simulink model "speed2"  (R2022b)
settings: Solver=VariableStepAuto  StartTime=0.0  StopTime=30  RelTol=1e-3
values from neighbouring files (symbols this model uses):
  Caf = 460.0    [VehCtrlMdelDictionary.sldd]    (also in trqvparameter.m = 460)
  Car = 440.0    [VehCtrlMdelDictionary.sldd]    (also in trqvparameter.m = 440)
  dwf = 1.2    [VehCtrlMdelDictionary.sldd]    (also in trqvparameter.m)
  Iz = 105.0    [VehCtrlMdelDictionary.sldd]    (also in trqvparameter.m = 105)
  Ki = 1.0    [VehCtrlMdelDictionary.sldd]    (also in trqvparameter.m = 20)
  Kp = 2.0    [VehCtrlMdelDictionary.sldd]    (also in trqvparameter.m = 30)
  lf = 0.761    [VehCtrlMdelDictionary.sldd]    (also in trqvparameter.m)
  lr = 0.831    [VehCtrlMdelDictionary.sldd]    (also in trqvparameter.m)
  m = 340.0    [VehCtrlMdelDictionary.sldd]    (also in trqvparameter.m = 340)
  Rt = 0.2    [VehCtrlMdelDictionary.sldd]    (also in trqvparameter.m)
libraries: simulink x12, Solver_SF x1
settings Model: Creator=12045  LastModifiedBy=12045

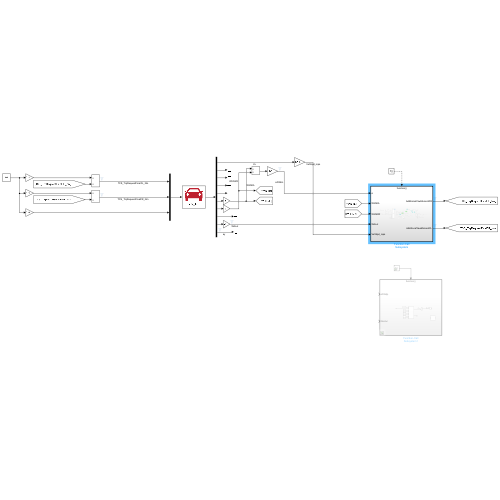
[thumbnail: Simulink's stored preview of the top-level diagram]
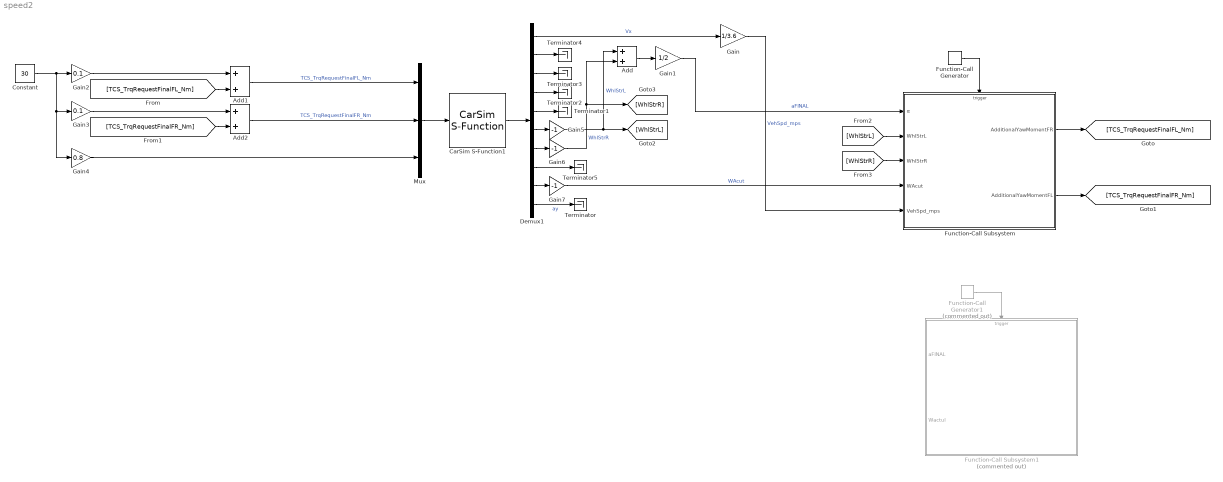
== system speed2 ==
  Add : Sum
  Add1 : Sum
  Add2 : Sum
  CarSim S-Function1 : Solver_SF/CarSim S-Function  Priority=1  SIMFILE=simfile.sim  Run_RTs=off  vs_state_ind=Run  StopMode_ind=Vehicle Model
  Constant : Constant  Value=30
  Demux1 : Demux  Outputs=10
  Function-Call Generator : simulink/Ports & Subsystems/Function-Call Generator  sample_time=0.01  numberOfIterations=1  DisallowWideOutput=off
  Function-Call Generator1 : simulink/Ports & Subsystems/Function-Call Generator  Commented=on  sample_time=0.01  numberOfIterations=1  DisallowWideOutput=off
  Function-Call Subsystem : Subsystem  TreatAsAtomicUnit=on
  Function-Call Subsystem1 : Subsystem  Commented=on  TreatAsAtomicUnit=on
  Gain : Gain  Gain=1/3.6
  Gain1 : Gain  Gain=1/2
  Gain2 : Gain  Gain=0.1
  Gain3 : Gain  Gain=0.1
  Gain4 : Gain  Gain=0.8
  Gain5 : Gain  Gain=-1
  Gain6 : Gain  Gain=-1
  Gain7 : Gain  Gain=-1
  Mux : Mux  Inputs=3
  Terminator{,1..5} (6 alike) : Terminator
  wires:
  Add2/1 -> Mux/2  "TCS_TrqRequestFinalFR_Nm"
  Add1/1 -> Mux/1  "TCS_TrqRequestFinalFL_Nm"
  Mux/1 -> CarSim S-Function1/1
  Function-Call Generator/1 -> Function-Call Subsystem/Trigger
  Gain6/1 -> Add/2, [WhlStrR]  "WhlStrR"
  Gain7/1 -> Function-Call Subsystem/4(WAcut)  "WAcut"
  Demux1/6 -> Gain5/1
  Demux1/7 -> Gain6/1
  Demux1/9 -> Gain7/1
  Gain5/1 -> [WhlStrL], Add/1  "WhlStrL"
  CarSim S-Function1/1 -> Demux1/1
  Demux1/10 -> Terminator/1  "ay"
  Demux1/1 -> Gain/1  "Vx"
  Add/1 -> Gain1/1
  Function-Call Subsystem/1(AdditionalYawMomentFR) -> [TCS_TrqRequestFinalFL_Nm]
  Function-Call Subsystem/2(AdditionalYawMomentFL) -> [TCS_TrqRequestFinalFR_Nm]
  [WhlStrL] -> Function-Call Subsystem/2(WhlStrL)
  [WhlStrR] -> Function-Call Subsystem/3(WhlStrR)
  Demux1/5 -> Terminator1/1
  Demux1/4 -> Terminator2/1
  Demux1/3 -> Terminator3/1
  Demux1/2 -> Terminator4/1
  Demux1/8 -> Terminator5/1
  Constant/1 -> Gain4/1, Gain3/1, Gain2/1
  Gain2/1 -> Add1/1
  [TCS_TrqRequestFinalFL_Nm] -> Add1/2
  Gain3/1 -> Add2/1
  [TCS_TrqRequestFinalFR_Nm] -> Add2/2
  Gain4/1 -> Mux/3
  Gain/1 -> Function-Call Subsystem/5(VehSpd_mps)  "VehSpd_mps"
  Gain1/1 -> Function-Call Subsystem/1(α)  "aFINAL"
  Function-Call Generator1/1 -> Function-Call Subsystem1/Trigger

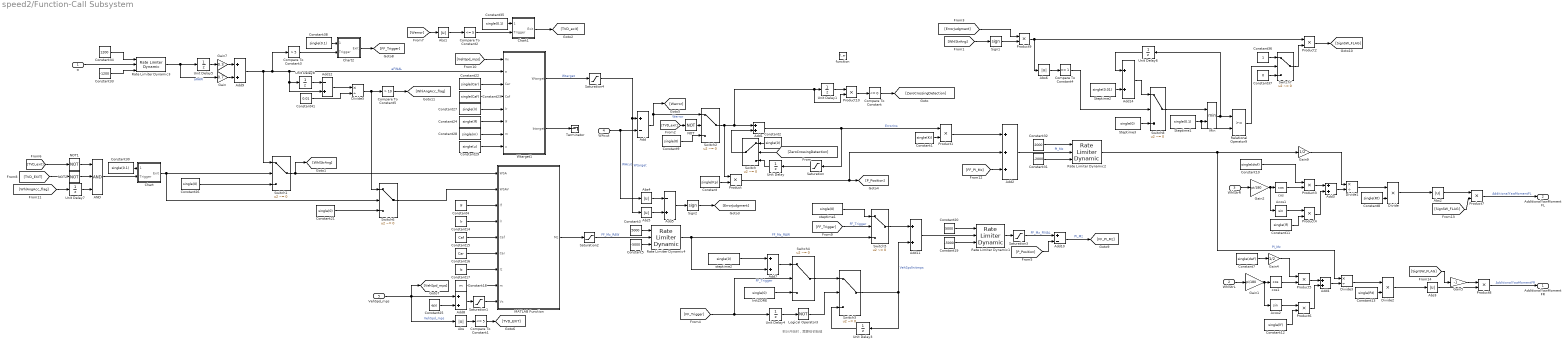
== system speed2/Function-Call Subsystem ==
  note: 积分开始时，需要给初始值
  α : Inport
  WhlStrL : Inport  Port=2
  WhlStrR : Inport  Port=3
  WAcut : Inport  Port=4
  VehSpd_mps : Inport  Port=5
  function : TriggerPort  TriggerType=function-call  VariantControl=(inherit)
  AND : Logic  Inputs=3  AllPortsSameDT=off  OutDataTypeStr=boolean
  Abs{,1..6} (7 alike) : Abs  SaturateOnIntegerOverflow=off
  Acos1 : Trigonometry
  Acos2 : Trigonometry
  Add : Sum  Inputs=+-
  Add{1,3..4,7..9,11,14} (8 alike) : Sum
  Add10 : Sum  Inputs=+-
  Add12 : Sum  Inputs=-+
  Add2 : Sum  Inputs=+++
  Add5 : Sum  Inputs=-+
  Chart : Stateflow chart  TreatAsAtomicUnit=on
  Chart1 : Stateflow chart  TreatAsAtomicUnit=on
  Chart2 : Stateflow chart  TreatAsAtomicUnit=on
  Compare To Constant : simulink/Logic and Bit Operations/Compare To Constant  relop=<=  const=0  OutDataTypeStr=boolean
  Compare To Constant1 : simulink/Logic and Bit Operations/Compare To Constant  relop=<=  const=5  OutDataTypeStr=boolean
  Compare To Constant2 : simulink/Logic and Bit Operations/Compare To Constant  relop=<=  const=5  OutDataTypeStr=boolean
  Compare To Constant3 : simulink/Logic and Bit Operations/Compare To Constant  relop=>  const=5  OutDataTypeStr=boolean
  Compare To Constant4 : simulink/Logic and Bit Operations/Compare To Constant  relop===  const=1  OutDataTypeStr=boolean
  Compare To Constant5 : simulink/Logic and Bit Operations/Compare To Constant  relop=>  const=10  OutDataTypeStr=boolean
  Constant : Constant  Value=single(Kp)
  Constant1 : Constant  Value=single(Ki)
  Constant10 : Constant  Value=single(dwf)
  Constant11 : Constant  Value=single(lf)
  Constant12 : Constant  Value=single(lf)
  Constant13 : Constant  Value=single(Rt)
  Constant14 : Constant  Value=lr
  Constant15 : Constant  Value=Caf
  Constant16 : Constant  Value=Car
  Constant17 : Constant  Value=Iz
  Constant18 : Constant  Value=m
  Constant19 : Constant  Value=-5000
  Constant{2,9,21,26} (4 alike) : Constant  Value=single(0)
  Constant20 : Constant  Value=5000
  Constant22 : Constant  Value=single(Car)
  Constant23 : Constant  Value=single(Caf)
  Constant24 : Constant  Value=single(lf)
  Constant25 : Constant  Value=eps
  Constant27 : Constant  Value=single(lr)
  Constant28 : Constant  Value=single(m)
  Constant29 : Constant  Value=single(u)
  Constant3 : Constant  Value=5000
  Constant30 : Constant  Value=single(0.1)
  Constant31 : Constant  Value=-2000
  Constant32 : Constant  Value=2000
  Constant33 : Constant  Value=-1200
  Constant34 : Constant  Value=1200
  Constant35 : Constant  Value=single(0.1)
  Constant36 : Constant
  Constant37 : Constant  Value=0
  Constant38 : Constant  Value=single(0.1)
  Constant4 : Constant  Value=lf
  Constant41 : Constant  Value=0.01
  Constant5 : Constant  Value=-5000
  Constant7 : Constant  Value=single(dwf)
  Constant8 : Constant  Value=single(Rt)
  Divide : Product  Inputs=**
  Divide1 : Product  Inputs=*/
  Divide2 : Product  Inputs=**
  Divide3 : Product  Inputs=*/
  Divide5 : Product  Inputs=*/
  Gain : Gain  Gain=0.7
  Gain1 : Gain  Gain=pi/180
  Gain2 : Gain  Gain=pi/180
  Gain4 : Gain  Gain=1/2
  Gain5 : Gain  Gain=-1
  Gain7 : Gain  Gain=0.3
  Gain9 : Gain  Gain=1/2
  InitZORE : Constant  Value=single(0)
  Logical Operator3 : Logic  Operator=NOT  AllPortsSameDT=off  OutDataTypeStr=boolean
  MATLAB Function : MATLAB Function  TreatAsAtomicUnit=on
  Min : MinMax  Inputs=2
  NOT : Logic  Operator=NOT  AllPortsSameDT=off  OutDataTypeStr=boolean
  NOT1 : Logic  Operator=NOT  AllPortsSameDT=off  OutDataTypeStr=boolean
  NOT2 : Logic  Operator=NOT  AllPortsSameDT=off  OutDataTypeStr=boolean
  Product{,1..10} (11 alike) : Product
  Rate Limiter Dynamic{1..4} (4 alike) : simulink/Discontinuities/Rate Limiter Dynamic
  Relational Operator9 : RelationalOperator  OutDataTypeStr=boolean  RndMeth=Simplest  InputSameDT=off
  Saturation : Saturate  UpperLimit=10  LowerLimit=-10
  Saturation1 : Saturate  UpperLimit=40  LowerLimit=0
  Saturation2 : Saturate  UpperLimit=5000  LowerLimit=-5000
  Saturation3 : Saturate  UpperLimit=300  LowerLimit=-300
  Saturation4 : Saturate  UpperLimit=50  LowerLimit=-50
  Sign1 : Signum
  Sign2 : Signum
  Steptime1 : Constant  Value=single(0.1)
  Steptime2 : Constant  Value=single(0.01)
  Steptime3 : Constant  Value=single(0)
  Switch{,1..8} (9 alike) : Switch  Criteria=u2 ~= 0  SaturateOnIntegerOverflow=off  InputSameDT=off
  Terminator : Terminator
  Unit Delay{,1,3..8} (8 alike) : UnitDelay  SampleTime=-1  HasFrameUpgradeWarning=on
  Wtarget1 : MATLAB Function  TreatAsAtomicUnit=on
  cos : Trigonometry  Operator=cos
  cos1 : Trigonometry  Operator=cos
  steptime1 : Constant  Value=single(0)
  steptime2 : Constant  Value=single(0)
  AdditionalYawMomentFR : Outport
  AdditionalYawMomentFL : Outport  Port=2
  wires:
  Wtarget1/1(Wtarget) -> Saturation4/1  "Wtarget"
  WAcut/1 -> Abs4/1, Add/2  "WAcut"
  Add/1 -> [Werror], Switch2/1  "Werror"
  Constant/1 -> Product/2
  Add1/1 -> Product1/1, Saturation/1  "ErrorIns"
  Constant1/1 -> Product1/2
  Product1/1 -> Add2/1
  Product/1 -> Add2/2, [P_Position]
  Saturation/1 -> Unit Delay/1
  Switch/1 -> Add1/2
  Constant2/1 -> Switch/1
  Unit Delay/1 -> Switch/3
  Compare To Constant/1 -> [ZeroCrossingDetection]
  [ZeroCrossingDetection] -> Switch/2
  Constant8/1 -> Divide/2
  Abs1/1 -> Compare To Constant2/1
  Switch2/1 -> Product10/2, Unit Delay1/1, Add1/1, Product/1
  [TVD_exit] -> NOT/1
  NOT/1 -> Switch2/2
  Constant9/1 -> Switch2/3
  WhlStrR/1 -> Gain2/1
  Gain2/1 -> Acos1/1, cos/1
  cos/1 -> Product3/2
  Constant10/1 -> Product3/1
  Product3/1 -> Add3/1
  Acos1/1 -> Product4/1
  Constant11/1 -> Product4/2
  Product4/1 -> Add3/2
  Add3/1 -> Divide1/2
  Divide1/1 -> Divide/1
  Divide/1 -> Abs2/1
  Divide3/1 -> Divide2/1
  Add4/1 -> Divide3/2
  Product6/1 -> Add4/2
  Constant12/1 -> Product6/2
  Acos2/1 -> Product6/1
  Product5/1 -> Add4/1
  Gain4/1 -> Product5/1
  cos1/1 -> Product5/2
  Constant7/1 -> Gain4/1
  Gain1/1 -> cos1/1, Acos2/1
  WhlStrL/1 -> Gain1/1
  Rate Limiter Dynamic2/1 -> Divide3/1, Gain9/1  "PI_Mz"
  Constant13/1 -> Divide2/2
  Divide2/1 -> Abs3/1
  Abs2/1 -> Product7/1
  Abs3/1 -> Product8/2
  Sign2/1 -> [ErrorJudgment]
  Sign1/1 -> Product9/2
  [ErrorJudgment] -> Product9/1
  Product9/1 -> Product2/1, Abs6/1
  Gain5/1 -> Product8/1
  Abs4/1 -> Add5/1
  Abs5/1 -> Add5/2
  Add5/1 -> Sign2/1
  Unit Delay1/1 -> Product10/1
  Product10/1 -> Compare To Constant/1
  Constant4/1 -> MATLAB Function/3(lf)
  Constant14/1 -> MATLAB Function/4(lr)
  Constant15/1 -> MATLAB Function/5(Caf)
  Constant16/1 -> MATLAB Function/6(Car)
  Constant17/1 -> MATLAB Function/7(Iz)
  Constant18/1 -> MATLAB Function/8(m)
  VehSpd_mps/1 -> Add8/1, Abs/1, [VehSpd_mps]  "VehSpd_mps"
  Switch1/1 -> [WhlStrAng], MATLAB Function/1(WSA)
  [WhlStrAng] -> Sign1/1
  Logical Operator3/1 -> Switch3/2
  steptime2/1 -> Add7/1
  Switch3/1 -> Add11/2, Unit Delay3/1  "VehSpdInitmps"
  Unit Delay4/1 -> Logical Operator3/1
  [FF_Trigger] -> Switch4/2, Unit Delay4/1  "FF_Trigger"
  Unit Delay3/1 -> Switch3/3
  Switch4/1 -> Switch3/1
  InitZORE/1 -> Switch4/3
  Add7/1 -> Switch4/1
  Add8/1 -> Saturation1/1
  Constant25/1 -> Add8/2
  Saturation1/1 -> MATLAB Function/9(Vx)
  [P_Position] -> Add10/2
  MATLAB Function/1(Mz) -> Saturation2/1
  Constant26/1 -> Switch1/3
  Rate Limiter Dynamic3/1 -> Unit Delay5/1, Gain/1  "aRAW"
  [TVD_exit] -> NOT1/1
  NOT1/1 -> AND/1
  [Werror] -> Abs1/1
  Rate Limiter Dynamic4/1 -> Add7/2, Switch5/3  "FF_Mz_RAW"
  Abs/1 -> Compare To Constant1/1
  Compare To Constant1/1 -> [TVD_EXIT]
  [TVD_EXIT] -> NOT2/1
  NOT2/1 -> AND/2
  Chart/1(Exit) -> Switch6/2, Switch1/2
  [FF_Trigger] -> Switch5/2  "FF_Trigger"
  Switch5/1 -> Add11/1
  steptime1/1 -> Switch5/1
  Add11/1 -> Rate Limiter Dynamic1/2
  Constant19/1 -> Rate Limiter Dynamic1/3
  Rate Limiter Dynamic1/1 -> Saturation3/1
  Constant20/1 -> Rate Limiter Dynamic1/1
  Saturation3/1 -> Add10/1  "FF_Mz_FINAL"
  Constant21/1 -> Switch6/3
  Switch6/1 -> MATLAB Function/2(WSAV)
  Constant22/1 -> Wtarget1/3(Car)
  Constant28/1 -> Wtarget1/7(m)
  Constant27/1 -> Wtarget1/5(lr)
  Constant29/1 -> Wtarget1/8(u)
  Constant24/1 -> Wtarget1/6(lf)
  Constant23/1 -> Wtarget1/4(Caf)
  [VehSpd_mps] -> Wtarget1/1(Vx)
  Wtarget1/2(btarget) -> Terminator/1
  Saturation4/1 -> Abs5/1, Add/1  "Wtarget"
  AND/1 -> Chart/2(Trigger)
  Constant30/1 -> Chart/1(CountTime)
  Constant32/1 -> Rate Limiter Dynamic2/1
  Constant31/1 -> Rate Limiter Dynamic2/3
  Add2/1 -> Rate Limiter Dynamic2/2  "PI_Mz"
  Unit Delay5/1 -> Gain7/1
  Add9/1 -> Compare To Constant3/1, Add12/2, Unit Delay8/1, Wtarget1/2(a), Switch1/1  "aFINAL"
  Gain/1 -> Add9/2
  Gain7/1 -> Add9/1
  α/1 -> Rate Limiter Dynamic3/2
  Constant33/1 -> Rate Limiter Dynamic3/3
  Constant34/1 -> Rate Limiter Dynamic3/1
  Product7/1 -> AdditionalYawMomentFL/1  "AdditionalYawMomentFL"
  Product8/1 -> AdditionalYawMomentFR/1  "AdditionalYawMomentFR"
  Abs6/1 -> Compare To Constant4/1
  Relational Operator9/1 -> Switch7/2
  Switch7/1 -> Product2/2
  Constant36/1 -> Switch7/1
  Constant37/1 -> Switch7/3
  Min/1 -> Relational Operator9/1, Unit Delay6/1
  Compare To Constant4/1 -> Switch8/2
  Add14/1 -> Switch8/1
  Unit Delay6/1 -> Add14/1
  Steptime3/1 -> Switch8/3
  Switch8/1 -> Min/1
  Steptime2/1 -> Add14/2
  Steptime1/1 -> Relational Operator9/2, Min/2
  [FF_PI_Mz] -> Add2/3
  Product2/1 -> [SignSW_FLAG]
  [SignSW_FLAG] -> Product7/2
  [SignSW_FLAG] -> Gain5/1
  Gain9/1 -> Divide1/1
  Constant35/1 -> Chart1/1(CountTime)
  Compare To Constant2/1 -> Chart1/2(Trigger)
  Chart1/1(Exit) -> [TVD_exit]
  Compare To Constant3/1 -> Chart2/2(Trigger)
  Constant38/1 -> Chart2/1(CountTime)
  Chart2/1(Exit) -> [FF_Trigger]
  Add10/1 -> [FF_PI_Mz]  "PI_Mz"
  Compare To Constant5/1 -> [WhlAngAcc_flag]
  [WhlAngAcc_flag] -> Unit Delay7/1
  Unit Delay7/1 -> AND/3
  Constant41/1 -> Divide5/2
  Add12/1 -> Divide5/1
  Unit Delay8/1 -> Add12/1
  Divide5/1 -> Switch6/1, Compare To Constant5/1
  Saturation2/1 -> Rate Limiter Dynamic4/2  "FF_Mz_RAW"
  Constant3/1 -> Rate Limiter Dynamic4/1
  Constant5/1 -> Rate Limiter Dynamic4/3

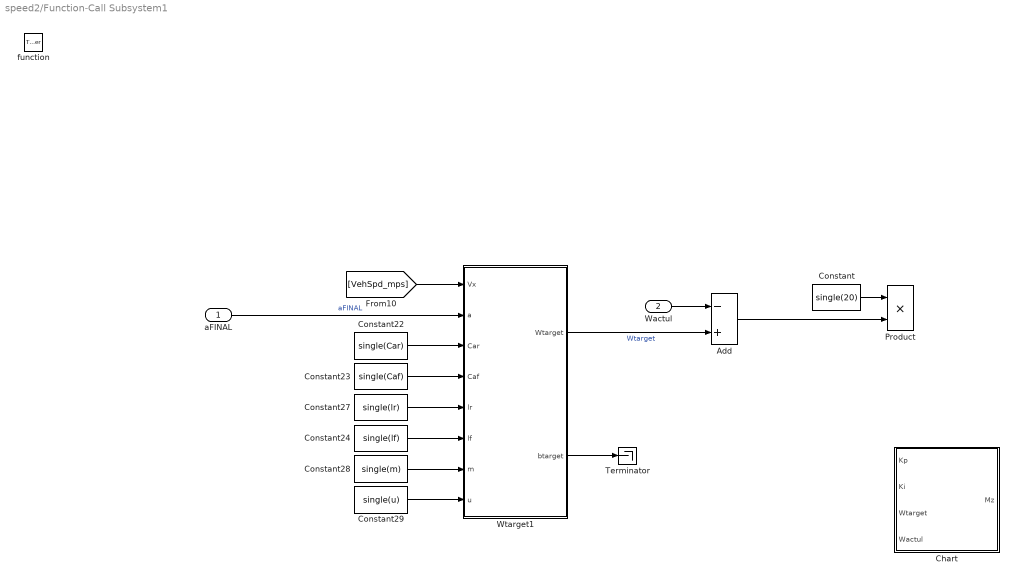
== system speed2/Function-Call Subsystem1 ==
  aFINAL : Inport
  Wactul : Inport  Port=2
  function : TriggerPort  TriggerType=function-call  VariantControl=(inherit)
  Add : Sum  Inputs=-+
  Chart : Stateflow chart  TreatAsAtomicUnit=on
  Constant : Constant  Value=single(20)
  Constant22 : Constant  Value=single(Car)
  Constant23 : Constant  Value=single(Caf)
  Constant24 : Constant  Value=single(lf)
  Constant27 : Constant  Value=single(lr)
  Constant28 : Constant  Value=single(m)
  Constant29 : Constant  Value=single(u)
  Product : Product
  Terminator : Terminator
  Wtarget1 : MATLAB Function  TreatAsAtomicUnit=on
  wires:
  Constant29/1 -> Wtarget1/8(u)
  Constant23/1 -> Wtarget1/4(Caf)
  Constant27/1 -> Wtarget1/5(lr)
  Constant28/1 -> Wtarget1/7(m)
  [VehSpd_mps] -> Wtarget1/1(Vx)
  aFINAL/1 -> Wtarget1/2(a)  "aFINAL"
  Constant24/1 -> Wtarget1/6(lf)
  Constant22/1 -> Wtarget1/3(Car)
  Wtarget1/1(Wtarget) -> Add/2  "Wtarget"
  Wtarget1/2(btarget) -> Terminator/1
  Wactul/1 -> Add/1
  Add/1 -> Product/2
  Constant/1 -> Product/1

== stateflow chart speed2/Function-Call Subsystem/Chart ==
  state Trigger
    en:
    x = x + 0.01;
    Exit=0;
  state Out
    en:
    Exit=1;
    x=0;
  state InterState
    en:
    x=0;
  Trigger -> Trigger [order 2] : [Trigger&&x<CountTime]
  Trigger -> Out [order 3] : [x>=CountTime]
  (default) -> Trigger
  Out -> Trigger : [~Trigger]
  InterState -> Trigger : [Trigger]
  Trigger -> InterState [order 1] : [x<CountTime&&~Trigger]
  data: CountTime input; Trigger input; Exit output; x local =0

== stateflow chart speed2/Function-Call Subsystem/Chart1 ==
  state Trigger
    en:
    x = x + 0.01;
    Exit=0;
  state Out
    en:
    Exit=1;
    x=0;
  state InterState
    en:
    x=0;
  Trigger -> Trigger [order 2] : [Trigger&&x<CountTime]
  Trigger -> Out [order 3] : [x>=CountTime]
  (default) -> Trigger
  Out -> Trigger : [~Trigger]
  InterState -> Trigger : [Trigger]
  Trigger -> InterState [order 1] : [x<CountTime&&~Trigger]
  data: CountTime input; Trigger input; Exit output; x local =0

== stateflow chart speed2/Function-Call Subsystem/Chart2 ==
  state Trigger
    en:
    x = x + 0.01;
    Exit=0;
  state Out
    en:
    Exit=1;
    x=0;
  state InterState
    en:
    x=0;
  Trigger -> Trigger [order 2] : [Trigger&&x<CountTime]
  Trigger -> Out [order 3] : [x>=CountTime]
  (default) -> Trigger
  Out -> Trigger : [~Trigger]
  InterState -> Trigger : [Trigger]
  Trigger -> InterState [order 1] : [x<CountTime&&~Trigger]
  data: CountTime input; Trigger input; Exit output; x local =0

== stateflow chart speed2/Function-Call Subsystem1/Chart ==
  (default) -> (junction 21)
  (junction 21) -> (junction 23) : {Werror=Wtarget-Wactul}
  (junction 23) -> (junction 25) [order 1]
  (junction 23) -> (junction 38) [order 2] : {K=Kp*Werror}
  (junction 25) -> (junction 27)
  (junction 27) -> (junction 29) : {I_Pres=I_Prev+Werror*Ki}
  (junction 33) -> (junction 27) [order 1]
  (junction 29) -> (junction 31) : {Temp=I_Pres}
  (junction 31) -> (junction 33) : {I_Prev=Temp}
  (junction 33) -> (junction 36) [order 2] : {I=I_Pres}
  (junction 36) -> (junction 38)
  (junction 38) -> (junction 41) : {Mz=K+I}
  data: Kp input; Ki input; Wtarget input; Wactul input; Mz output =0; I_Prev local =0; I local; K local; Werror local; Temp local; I_Pres local

== matlab function speed2/Function-Call Subsystem1/Wtarget1 ==
  data: Vx input size=1; Wtarget output size=1; a input size=1; Car input size=1; Caf input size=1; lr input size=1; lf input size=1; m input; u input; btarget output
function [Wtarget,btarget] = fcn(Vx,a,Car,Caf,lr,lf,m,u)
Wdes = Vx*a/(lf+lr+(m*Vx*Vx*(lr*Car-lf*Caf)/Caf/Car/(lr+lf)/2));
Wu = 0.85*u*9.8/Vx;
%if abs(Wdes)<=Wu
Wtarget = Wdes;
%else
 %   Wtarget = Wu*sign(Wdes);
%end
bdes = (lr-lf*m*Vx*Vx/Car/(lf+lr)/2)*a/(lr+lf+m*Vx*Vx*(lr*Car-lf*Caf)/Car/Caf/(lf+lr)/2);
bu = atan(0.02*u*9.8);
if abs(bdes)<=bu
btarget = bdes;
else
    btarget = bu*sign(bdes);
end

== matlab function speed2/Function-Call Subsystem/Wtarget1 ==
  data: Vx input size=1; Wtarget output size=1; a input size=1; Car input size=1; Caf input size=1; lr input size=1; lf input size=1; m input; u input; btarget output
function [Wtarget,btarget] = fcn(Vx,a,Car,Caf,lr,lf,m,u)
Wdes = Vx*a/(lf+lr+(m*Vx*Vx*(lr*Car-lf*Caf)/Caf/Car/(lr+lf)/2));
Wu = 0.85*u*9.8/Vx;
%if abs(Wdes)<=Wu
Wtarget = Wdes;
%else
 %   Wtarget = Wu*sign(Wdes);
%end
bdes = (lr-lf*m*Vx*Vx/Car/(lf+lr)/2)*a/(lr+lf+m*Vx*Vx*(lr*Car-lf*Caf)/Car/Caf/(lf+lr)/2);
bu = atan(0.02*u*9.8);
if abs(bdes)<=bu
btarget = bdes;
else
    btarget = bu*sign(bdes);
end

== matlab function speed2/Function-Call Subsystem/MATLAB Function ==
  data: WSA input; Mz output; WSAV input; lf input; lr input; Caf input; Car input; Iz input; m input; Vx input
function Mz = fcn(WSA,WSAV,lf,lr,Caf,Car,Iz,m,Vx)

Mz = ((((lf*lf*Caf+lr*lr*Car)/Iz/Vx)*(-Caf/m/Vx)-((lf*Caf-lr*Car)/m/Vx/Vx-1)*(-lf*Caf/Iz))*Iz*WSA-(-Caf/m/Vx)*Iz*WSAV)/((lf*Caf-lr*Car)/m/Vx/Vx-1);
